simulink model "drone_model"  (R2024b)
settings: Solver=VariableStepAuto  StartTime=0.0  StopTime=10.0  RelTol=1e-3
values from neighbouring files (symbols this model uses):
  b = C_T*rho_A*D^4    (= 7.687659375e-05)    [drone_params.m]
  d = C_p*rho_A*D^5    (= 4.71742734375e-06)    [drone_params.m]
  g = 9.81    [drone_params.m]
  I_xx = 5144.434e-6    (= 0.005144434)    [drone_params.m]
  I_yy = 5144.434e-6    (= 0.005144434)    [drone_params.m]
  I_zz = 10289.036e-6    (= 0.010289036)    [drone_params.m]
  J_r = 15e-6    (= 1.5e-05)    [drone_params.m]
  l = 0.2    [drone_params.m]
  m = 0.568    [drone_params.m]
settings Model: Creator=andit  LastModifiedBy=andit

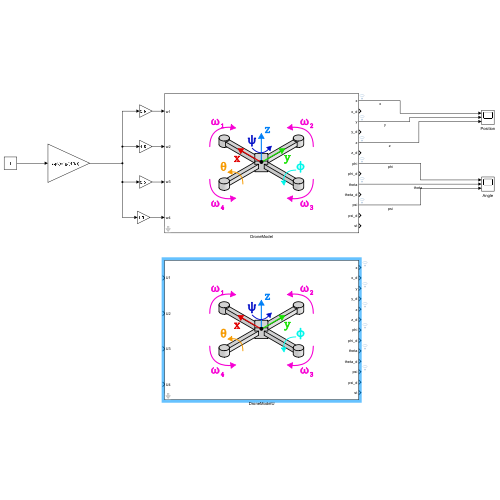
[thumbnail: Simulink's stored preview of the top-level diagram]
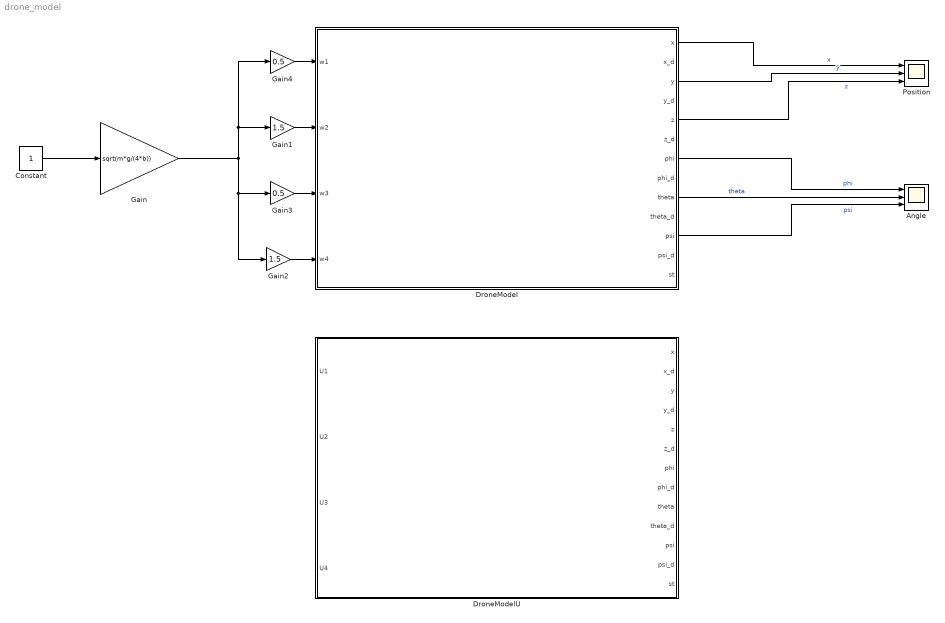
== system drone_model ==
  Angle : Scope  NumInputPorts=3
  Constant : Constant
  DroneModel : Subsystem  mask{m=m, g=g, l=l, I_xx=I_xx, I_yy=I_yy, I_zz=I_zz, J_r=J_r, b=b, d=d}
      mask prompts: m "mass"; l "length from rotor"; J_r "Motor Inertia J_r"; b "Thrust factor b"; d "Drag factor d"
      mask DialogControl THETA Prompt: Principle Moments of Inertia
      mask DialogControl PROPELLER Prompt: Propeller Coefficients
  DroneModelU : Subsystem  mask{m=m, g=g, l=l, I_xx=I_xx, I_yy=I_yy, I_zz=I_zz, J_r=J_r, b=b, d=d}
      mask prompts: m "mass"; l "length from rotor"; J_r "Motor Inertia J_r"; b "Thrust factor b"; d "Drag factor d"
      mask DialogControl THETA Prompt: Principle Moments of Inertia
      mask DialogControl PROPELLER Prompt: Propeller Coefficients
  Gain : Gain  Gain=sqrt(m*g/(4*b))
  Gain1 : Gain  Gain=1.5
  Gain2 : Gain  Gain=1.5
  Gain3 : Gain  Gain=0.5
  Gain4 : Gain  Gain=0.5
  Position : Scope  NumInputPorts=3
  wires:
  DroneModel/1(x) -> Position/1  "x"
  DroneModel/3(y) -> Position/2  "y"
  DroneModel/5(z) -> Position/3  "z"
  DroneModel/7(phi) -> Angle/1  "phi"
  DroneModel/9(theta) -> Angle/2  "theta"
  DroneModel/11(psi) -> Angle/3  "psi"
  Constant/1 -> Gain/1
  Gain/1 -> Gain3/1, Gain2/1, Gain1/1, Gain4/1
  Gain1/1 -> DroneModel/2(w2)
  Gain2/1 -> DroneModel/4(w4)
  Gain3/1 -> DroneModel/3(w3)
  Gain4/1 -> DroneModel/1(w1)

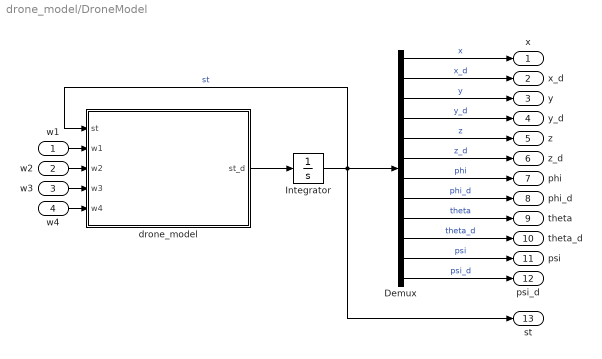
== system drone_model/DroneModel ==
  w1 : Inport
  w2 : Inport  Port=2
  w3 : Inport  Port=3
  w4 : Inport  Port=4
  Demux : Demux  Outputs=12
  Integrator : Integrator  InitialCondition=zeros(12,1)
  drone_model : MATLAB Function  TreatAsAtomicUnit=on
  x : Outport
  x_d : Outport  Port=2
  y : Outport  Port=3
  y_d : Outport  Port=4
  z : Outport  Port=5
  z_d : Outport  Port=6
  phi : Outport  Port=7
  phi_d : Outport  Port=8
  theta : Outport  Port=9
  theta_d : Outport  Port=10
  psi : Outport  Port=11
  psi_d : Outport  Port=12
  st : Outport  Port=13
  wires:
  drone_model/1(st_d) -> Integrator/1
  Demux/9 -> theta/1  "theta"
  w4/1 -> drone_model/5(w4)
  Integrator/1 -> st/1, Demux/1, drone_model/1(st)  "st"
  w3/1 -> drone_model/4(w3)
  Demux/7 -> phi/1  "phi"
  w2/1 -> drone_model/3(w2)
  w1/1 -> drone_model/2(w1)
  Demux/3 -> y/1  "y"
  Demux/11 -> psi/1  "psi"
  Demux/10 -> theta_d/1  "theta_d"
  Demux/2 -> x_d/1  "x_d"
  Demux/12 -> psi_d/1  "psi_d"
  Demux/6 -> z_d/1  "z_d"
  Demux/1 -> x/1  "x"
  Demux/8 -> phi_d/1  "phi_d"
  Demux/4 -> y_d/1  "y_d"
  Demux/5 -> z/1  "z"

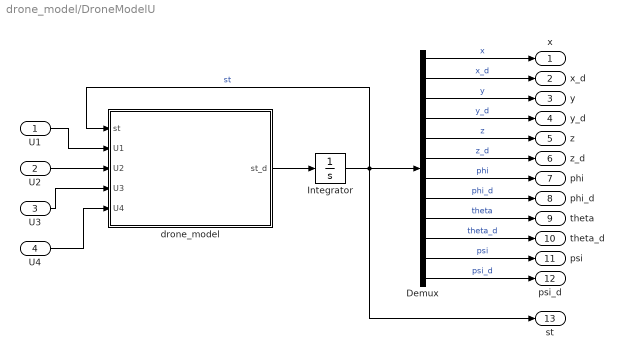
== system drone_model/DroneModelU ==
  U1 : Inport
  U2 : Inport  Port=2
  U3 : Inport  Port=3
  U4 : Inport  Port=4
  Demux : Demux  Outputs=12
  Integrator : Integrator  InitialCondition=zeros(12,1)
  drone_model : MATLAB Function  TreatAsAtomicUnit=on
  x : Outport
  x_d : Outport  Port=2
  y : Outport  Port=3
  y_d : Outport  Port=4
  z : Outport  Port=5
  z_d : Outport  Port=6
  phi : Outport  Port=7
  phi_d : Outport  Port=8
  theta : Outport  Port=9
  theta_d : Outport  Port=10
  psi : Outport  Port=11
  psi_d : Outport  Port=12
  st : Outport  Port=13
  wires:
  drone_model/1(st_d) -> Integrator/1
  Demux/9 -> theta/1  "theta"
  U4/1 -> drone_model/5(U4)
  Integrator/1 -> st/1, Demux/1, drone_model/1(st)  "st"
  U3/1 -> drone_model/4(U3)
  Demux/7 -> phi/1  "phi"
  U2/1 -> drone_model/3(U2)
  U1/1 -> drone_model/2(U1)
  Demux/3 -> y/1  "y"
  Demux/11 -> psi/1  "psi"
  Demux/10 -> theta_d/1  "theta_d"
  Demux/2 -> x_d/1  "x_d"
  Demux/12 -> psi_d/1  "psi_d"
  Demux/6 -> z_d/1  "z_d"
  Demux/1 -> x/1  "x"
  Demux/8 -> phi_d/1  "phi_d"
  Demux/4 -> y_d/1  "y_d"
  Demux/5 -> z/1  "z"

== matlab function drone_model/DroneModelU/drone_model ==
  data: st input; st_d output; U1 input; U2 input; U3 input; U4 input; m parameter; g parameter; l parameter; I_xx parameter; I_yy parameter; I_zz parameter; J_r parameter; b parameter; d parameter
function st_d = drone_model(st, U1, U2, U3, U4, m, g, l, I_xx, I_yy, I_zz, J_r, b, d)

% st = [x, x_d, y, y_d, z, z_d, phi, phi_d, theta, theta_d, psi, psi_d]

phi     = st(7);    phi_d   = st(8);
theta   = st(9);    theta_d = st(10);
psi     = st(11);   psi_d   = st(12);

Omega = 0;   % (i try neglecting gyroscopic effect)

x_dd = 1/m * (cos(phi)*sin(theta)*cos(psi) - sin(phi)*sin(psi))*U1;
y_dd = 1/m * (cos(phi)*sin(theta)*sin(psi) + sin(phi)*cos(psi))*U1;
z_dd = -g + 1/m * (cos(phi)*cos(theta))*U1;

phi_dd = 1/I_xx * (theta_d*psi_d*(I_zz-I_yy) - J_r*theta_d*Omega + l*U2);
theta_dd = 1/I_yy * (phi_d*psi_d*(I_xx-I_zz) + J_r*phi_d*Omega + l*U3);
psi_dd = 1/I_zz * (phi_d*theta_d*(I_yy-I_xx) + U4);

st_d = [st(2); x_dd; ...            % x_d, x_dd
        st(4); y_dd; ...            % y_d, y_dd
        st(6); z_dd; ...            % z_d, z_dd
        st(8); phi_dd; ...          % phi_d, phi_dd
        st(10); theta_dd; ...       % theta_d, theta_dd
        st(12); psi_dd];            % psi_d, psi_dd

== matlab function drone_model/DroneModel/drone_model ==
  data: st input; st_d output; w1 input; w2 input; w3 input; w4 input; m parameter; g parameter; l parameter; I_xx parameter; I_yy parameter; I_zz parameter; J_r parameter; b parameter; d parameter
function st_d = drone_model(st, w1, w2, w3, w4, m, g, l, I_xx, I_yy, I_zz, J_r, b, d)

% st = [x, x_d, y, y_d, z, z_d, phi, phi_d, theta, theta_d, psi, psi_d]

phi     = st(7);    phi_d   = st(8);
theta   = st(9);    theta_d = st(10);
psi     = st(11);   psi_d   = st(12);

U1 = b*(w1^2 + w2^2 + w3^2 + w4^2);     % total thrust
U2 = b*(w4^2 - w2^2);                   % Force diff for Roll
U3 = b*(w3^2 - w1^2);                   % Force diff for Pitch
U4 = d*(w2^2 + w4^2 - w1^2 - w3^2);     % Drag torque for Yaw
Omega = w1 - w2 + w3 - w4;              % Residual rotor speed

x_dd = 1/m * (cos(phi)*sin(theta)*cos(psi) - sin(phi)*sin(psi))*U1;
y_dd = 1/m * (cos(phi)*sin(theta)*sin(psi) + sin(phi)*cos(psi))*U1;
z_dd = -g + 1/m * (cos(phi)*cos(theta))*U1;

phi_dd = 1/I_xx * (theta_d*psi_d*(I_zz-I_yy) - J_r*theta_d*Omega + l*U2);
theta_dd = 1/I_yy * (phi_d*psi_d*(I_xx-I_zz) + J_r*phi_d*Omega + l*U3);
psi_dd = 1/I_zz * (phi_d*theta_d*(I_yy-I_xx) + U4);

st_d = [st(2); x_dd; ...            % x_d, x_dd
        st(4); y_dd; ...            % y_d, y_dd
        st(6); z_dd; ...            % z_d, z_dd
        st(8); phi_dd; ...          % phi_d, phi_dd
        st(10); theta_dd; ...       % theta_d, theta_dd
        st(12); psi_dd];            % psi_d, psi_dd
